simulink model "zad2"  (R2017b)
settings: Solver=VariableStepAuto  StartTime=0.0  StopTime=0  RelTol=1e-3
libraries: CPOiS_SourcesSinks x9, CPOiS_DataManipulation x4, CPOiS_HistogramOperations x3, CPOiS_General x1
settings Model: Creator=kstefanc  LastModifiedBy=kstefanc

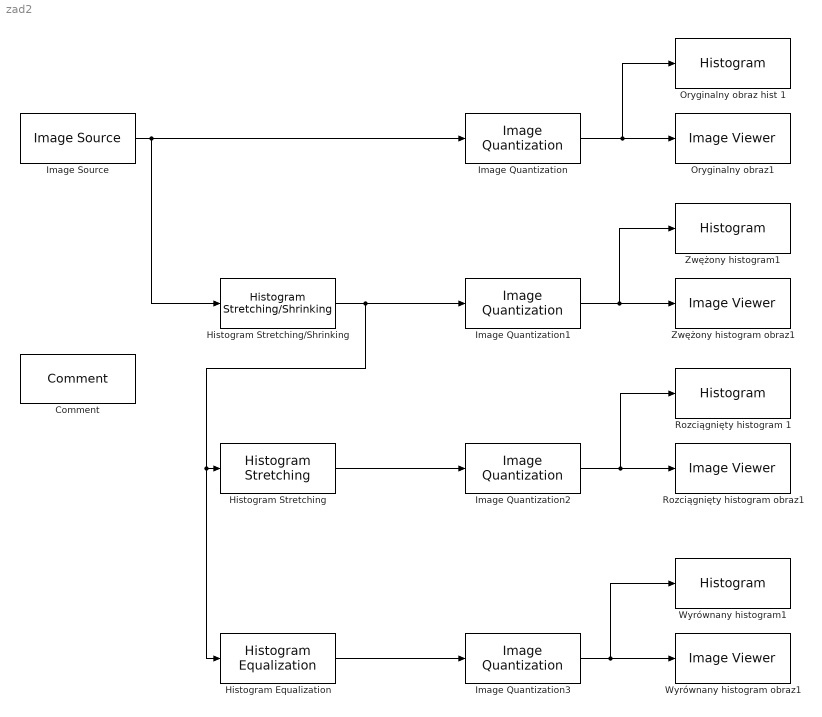
== system zad2 ==
  Comment : CPOiS_General/Comment
      settings: SourceProductName=CPOiS - Digital image and signal processing
  Histogram Stretching/Shrinking : CPOiS_HistogramOperations/Histogram Stretching//Shrinking  minimum=64  maximum=191
      settings: SourceProductName=CPOiS - Digital image and signal processing
  Histogram Equalization : CPOiS_HistogramOperations/Histogram Equalization
      settings: SourceProductName=CPOiS - Digital image and signal processing
  Histogram Stretching : CPOiS_HistogramOperations/Histogram Stretching
      settings: SourceProductName=CPOiS - Digital image and signal processing
  Image Quantization{,1..3} (4 alike) : CPOiS_DataManipulation/Image Quantization  LevelsNum=4
      settings: SourceProductName=CPOiS - Digital image and signal processing
  Image Source : CPOiS_SourcesSinks/Image Source  FileSelection=airport.png
      settings: SourceProductName=CPOiS - Digital image and signal processing
  Oryginalny obraz hist 1 : CPOiS_SourcesSinks/Histogram
      settings: SourceProductName=CPOiS - Digital image and signal processing
  Oryginalny obraz1 : CPOiS_SourcesSinks/Image Viewer
      settings: SourceProductName=CPOiS - Digital image and signal processing
  Rozciągnięty histogram 1 : CPOiS_SourcesSinks/Histogram
      settings: SourceProductName=CPOiS - Digital image and signal processing
  Rozciągnięty histogram obraz1 : CPOiS_SourcesSinks/Image Viewer
      settings: SourceProductName=CPOiS - Digital image and signal processing
  Wyrównany histogram obraz1 : CPOiS_SourcesSinks/Image Viewer
      settings: SourceProductName=CPOiS - Digital image and signal processing
  Wyrównany histogram1 : CPOiS_SourcesSinks/Histogram
      settings: SourceProductName=CPOiS - Digital image and signal processing
  Zwężony histogram obraz1 : CPOiS_SourcesSinks/Image Viewer
      settings: SourceProductName=CPOiS - Digital image and signal processing
  Zwężony histogram1 : CPOiS_SourcesSinks/Histogram
      settings: SourceProductName=CPOiS - Digital image and signal processing
  wires:
  Image Source/1 -> Histogram Stretching/Shrinking/1, Image Quantization/1
  Histogram Stretching/Shrinking/1 -> Histogram Equalization/1, Histogram Stretching/1, Image Quantization1/1
  Image Quantization3/1 -> Wyrównany histogram1/1, Wyrównany histogram obraz1/1
  Image Quantization2/1 -> Rozciągnięty histogram 1/1, Rozciągnięty histogram obraz1/1
  Image Quantization1/1 -> Zwężony histogram1/1, Zwężony histogram obraz1/1
  Image Quantization/1 -> Oryginalny obraz hist 1/1, Oryginalny obraz1/1
  Histogram Stretching/1 -> Image Quantization2/1
  Histogram Equalization/1 -> Image Quantization3/1
